simulink model "actionneur"  (R2019a)
settings: Solver=VariableStepAuto  StartTime=0.0  StopTime=10.0  RelTol=1e-3
settings Model: Creator=Nicolas Payeur  LastModifiedBy=Nicolas Payeur

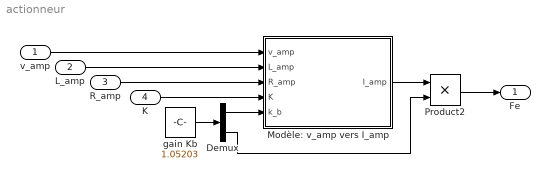
== system actionneur ==
  v_amp : Inport
  L_amp : Inport  Port=2
  R_amp : Inport  Port=3
  K : Inport  Port=4
  Demux : Demux  Outputs=2
  Modèle: v_amp vers I_amp : MATLAB Function  TreatAsAtomicUnit=on
  Product2 : Product
  gain Kb : Constant  Value=1.05203
  Fe : Outport  VectorParamsAs1DForOutWhenUnconnected=off
  wires:
  Product2/1 -> Fe/1
  Modèle: v_amp vers I_amp/1(I_amp) -> Product2/1
  v_amp/1 -> Modèle: v_amp vers I_amp/1(v_amp)
  R_amp/1 -> Modèle: v_amp vers I_amp/3(R_amp)
  L_amp/1 -> Modèle: v_amp vers I_amp/2(L_amp)
  gain Kb/1 -> Demux/1
  Demux/1 -> Modèle: v_amp vers I_amp/5(k_b)
  Demux/2 -> Product2/2
  K/1 -> Modèle: v_amp vers I_amp/4(K)

== matlab function actionneur/Modèle: v_amp vers I_amp ==
  data: v_amp input; I_amp output; L_amp input; R_amp input; K input; k_b input
function I_amp = fcn(v_amp, L_amp, R_amp, K, k_b)

I_amp = 1/(1+k_b/R_amp)*(K*exp(-R_amp*v_amp/L_amp)-L_amp/R_amp+...
    v_amp/R_amp);
end
